simulink model "warning_system"  (R2024b)
settings: Solver=FixedStepAuto  StartTime=0.0  StopTime=inf  FixedStep=TS_MODEL  RelTol=1e-3
InitFcn:
  | %run('config.m');
values from neighbouring files (symbols this model uses):
  ACCEL_RANGE = Simulink.Parameter    [config.m]
  DLPF_SETTING = Simulink.Parameter    [config.m]
  ENABLE_GYRO = Simulink.Parameter    [config.m]
undefined symbols (not defined in the file or in its folder): GYRO_RANGE, THRESHOLD_CAUTION, THRESHOLD_CRASHED, THRESHOLD_LANE_CHANGE, THRESHOLD_REST, TS_CORE, TS_GPS, TS_MPU, TS_PRINT, TS_READER, TS_WRITTER
libraries: arduinolib x5, dspstat3 x3, simulink x3
settings Model: DataDictionary=try.sldd  ExtModeTrigDuration=2  Creator=Nitesh  LastModifiedBy=Nitesh
settings SolverCC: AutoInsertRateTranBlk=on
settings OptimizationCC: EnhancedBackFolding=on  PassReuseOutputArgsAs=Individual arguments  ZeroExternalMemoryAtStartup=off  ZeroInternalMemoryAtStartup=off  MaxStackSize=64  OptimizeBlockOrder=speed  DifferentSizesBufferReuse=on  EfficientTunableParamExpr=on
settings DebuggingCC: ParameterTunabilityLossMsg=error
settings HardwareCC: ProdBitPerPointer=32  ProdBitPerSizeT=32  ProdBitPerPtrDiffT=32  ProdLargestAtomicInteger=Long  ProdLargestAtomicFloat=Double  ProdWordSize=32  ProdHWDeviceType=ARM Compatible->ARM Cortex
settings RTWCC: Description=Embedded Coder  SystemTargetFile=ert.tlc  HardwareBoard=ESP32-WROOM(Arduino Compatible)  TLCOptions="-aInlineSetEventsForThisBaseRateFcn=TLC_FALSE -aSuppressMultiTaskScheduler=TLC_FALSE  -aRateBasedStepFcn=0"  GenCodeOnly=on  PackageGeneratedCodeAndArtifacts=on  TemplateMakefile=ert_default_tmf  Toolchain=ESP32  GenerateCodeMetricsReport=on
settings CodeAppCC: ForceParamTrailComments=on  IgnoreCustomStorageClasses=off  MaxIdLength=51  OperatorAnnotations=on  SimulinkDataObjDesc=on  SFDataObjDesc=on  InsertBlockDesc=on
settings ERTTargetCC: MultiwordLength=2048  DynamicStringBufferSize=2048  InferredTypesCompatibility=on  SupportContinuousTime=on  SupportNonInlinedSFcns=on  SupportVariableSizeSignals=on  ExtModeTransport=3  ExtModeStaticAlloc=on  ExtModeAutomaticAllocSize=off  ExtModeStaticAllocSize=65536  ExtModeMexFile=ext_xcp  ExtModeIntrfLevel=Level2 - Open  InlinedParameterPlacement=Hierarchical

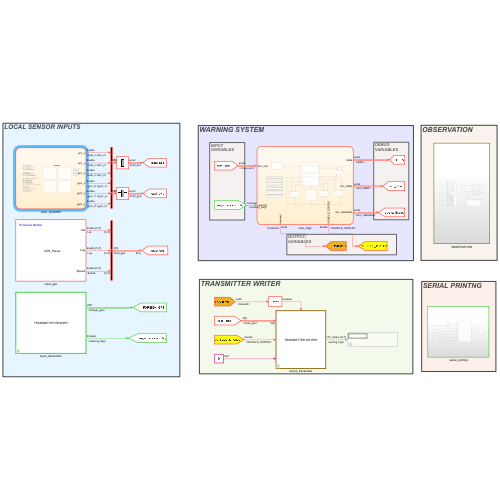
[thumbnail: Simulink's stored preview of the top-level diagram]
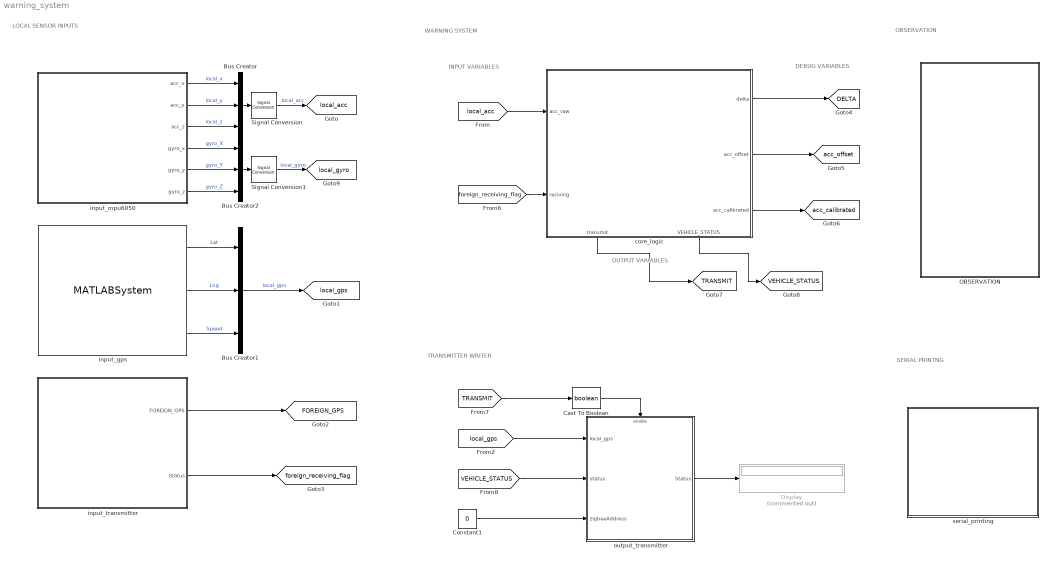
== system warning_system ==
  note: SERIAL PRINTNG
  note: DEBUG
      | VARIABLES
  note: OBSERVATION
  note: TRANSMITTER WRITER
  note: WARNING SYSTEM
  note: LOCAL SENSOR INPUTS
  note: OUTPUT
      | VARIABLES
  note: INPUT
      | VARIABLES
  " serial_printing" : Subsystem
      settings: RTWFileNameOpts=Use subsystem name
  Bus Creator : BusCreator  Inputs=3
  Bus Creator1 : BusCreator  Inputs=3
  Bus Creator2 : BusCreator  Inputs=3
  Cast To Boolean : DataTypeConversion  OutDataTypeStr=boolean  SaturateOnIntegerOverflow=off  RndMeth=Floor
  Constant1 : Constant  Value=0  OutDataTypeStr=half
  Display : Display  Commented=on
  OBSERVATION : Subsystem
  Signal Conversion : SignalConversion  ConversionOutput=Nonvirtual bus  OutDataTypeStr=Bus: accel  OverrideOpt=off
  Signal Conversion1 : SignalConversion  ConversionOutput=Nonvirtual bus  OutDataTypeStr=Bus: accel  OverrideOpt=off
  core_logic : Stateflow chart  TreatAsAtomicUnit=on  SystemSampleTime=TS_CORE
      settings: RTWSystemCode=Reusable function  RTWFileNameOpts=Use subsystem name  PortSchema="{\"entries\":[{\"content\":{\"sides\":[{\"content\":{\"connectorIds\":[\"In2\",\"In1\"]},\"type\":\"ConnectorPlacement.EquallySpacedRectSide\",\"uuid\":\"ee7c9145-97fe-42bf-b38f-25095debb339\"},{\"content\":{\"connectorIds\":[\"Out2\",\"Out3\",\"Out4\"],\"side\":\"RIGHT\"},\"type\":\"ConnectorPlacement.EquallySpacedRectSide\",\"uuid\":\"6ad3cc48-74a8-47e1-8b84-b3331846d199\"},{\"content\":{\"side\":\"TOP\"},\"type\":\"ConnectorPlacement.EquallySpacedRectSide\",\"uuid\":\"0e80e778-40c2-414e-b172-27c343627a22\"},{\"content\":{\"connectorIds\":[\"Out1\",\"Out5\"],\"side\":\"BOTTOM\"},\"type\":\"ConnectorPlacement.EquallySpacedRectSide\",\"uuid\":\"8c076511-fb77-4abd-9a6c-f32e2686fd08\"}]},\"type\":\"ConnectorPlacement.EquallySpacedConnector\",\"uuid\":\"44f6d062-1c8f-4774-b93e-5476bfb914ed\"}],\"packageUris\":[\"http://schema.mathworks.com/mf0/Connector/R2020b\"],\"version\":\"1.0\"}"
  input_gps : MATLABSystem  System=GPS_Parser  SampleTime=TS_GPS
      mask Type: GPS_Parser
      mask Display:
      | color('white');plot([100,100,100,100]*1,[100,100,100,100]*1);plot([100,100,100,100]*0,[100,100,100,100]*0);color('blue');text(38, 92, 'IO Device Builder','horizontalAlignment', 'right');
      | color('black');text(52,50,' GPS_Parser','horizontalAlignment','center');
      | port_label('output',1,'Lat');port_label('output',2,'Lng');port_label('output',3,'Speed');
  input_mpu6050 : Stateflow chart  TreatAsAtomicUnit=on  SystemSampleTime=TS_MPU
      settings: RTWSystemCode=Reusable function  RTWFileNameOpts=Use subsystem name  PortSchema="{\"entries\":[{\"content\":{\"sides\":[{\"content\":{},\"type\":\"ConnectorPlacement.EquallySpacedRectSide\",\"uuid\":\"e0cad0cf-2ed8-4cf7-bff6-6ed2feffa650\"},{\"content\":{\"connectorIds\":[\"Out1\",\"Out3\",\"Out2\",\"Out4\",\"Out5\",\"Out6\"],\"side\":\"RIGHT\"},\"type\":\"ConnectorPlacement.EquallySpacedRectSide\",\"uuid\":\"9c27c799-2435-4d39-8ba1-4c3814f68cde\"},{\"content\":{\"side\":\"TOP\"},\"type\":\"ConnectorPlacement.EquallySpacedRectSide\",\"uuid\":\"52d11aab-2c42-4a19-9ee0-cf61f3e3e234\"}]},\"type\":\"ConnectorPlacement.EquallySpacedConnector\",\"uuid\":\"b37ebc91-bb9d-4b35-9b01-6a26108d89d3\"}],\"packageUris\":[\"http://schema.mathworks.com/mf0/Connector/R2020b\"],\"version\":\"1.0\"}"
  input_transmitter : Subsystem  TreatAsAtomicUnit=on
      settings: RTWFileNameOpts=Use subsystem name
      mask Display: disp('TRANSMITTER READER');
  output_transmitter : Subsystem
      settings: RTWFileNameOpts=Use subsystem name
      mask Display: disp('TRANSMITTER WRITER');
  tag scope: DELTA=global, FOREIGN_GPS=global, TRANSMIT=global, VEHICLE_STATUS=global, acc_calibrated=global, acc_offset=global, foreign_receiving_flag=global, local_acc=global, local_gps=global, local_gyro=global
  wires:
  input_mpu6050/1(acc_x) -> Bus Creator/1  "local_x"
  input_mpu6050/3(acc_y) -> Bus Creator/2  "local_y"
  input_mpu6050/2(acc_z) -> Bus Creator/3  "local_z"
  Bus Creator/1 -> Signal Conversion/1
  [local_acc] -> core_logic/2(acc_raw)
  Bus Creator1/1 -> [local_gps]  "local_gps"
  Constant1/1 -> output_transmitter/3(zigbeeAddress)
  input_transmitter/1(FOREIGN_GPS) -> [FOREIGN_GPS]
  output_transmitter/1(Status) -> Display/1
  input_transmitter/2(Status) -> [foreign_receiving_flag]
  [foreign_receiving_flag] -> core_logic/1(reciving)
  core_logic/2(delta) -> [DELTA]
  core_logic/3(acc_offset) -> [acc_offset]
  core_logic/4(acc_calibrated) -> [acc_calibrated]
  core_logic/5(VEHICLE_STATUS) -> [VEHICLE_STATUS]
  core_logic/1(transmit) -> [TRANSMIT]
  [VEHICLE_STATUS] -> output_transmitter/2(status)
  [TRANSMIT] -> Cast To Boolean/1
  Cast To Boolean/1 -> output_transmitter/Enable
  input_mpu6050/4(gyro_x) -> Bus Creator2/1  "gyro_X"
  input_mpu6050/5(gyro_y) -> Bus Creator2/2  "gyro_Y"
  input_mpu6050/6(gyro_z) -> Bus Creator2/3  "gyro_Z"
  Bus Creator2/1 -> Signal Conversion1/1
  [local_gps] -> output_transmitter/1(local_gps)
  input_gps/1 -> Bus Creator1/1  "Lat"
  input_gps/2 -> Bus Creator1/2  "Lng"
  input_gps/3 -> Bus Creator1/3  "Speed"
  Signal Conversion/1 -> [local_acc]  "local_acc"
  Signal Conversion1/1 -> [local_gyro]  "local_gyro"

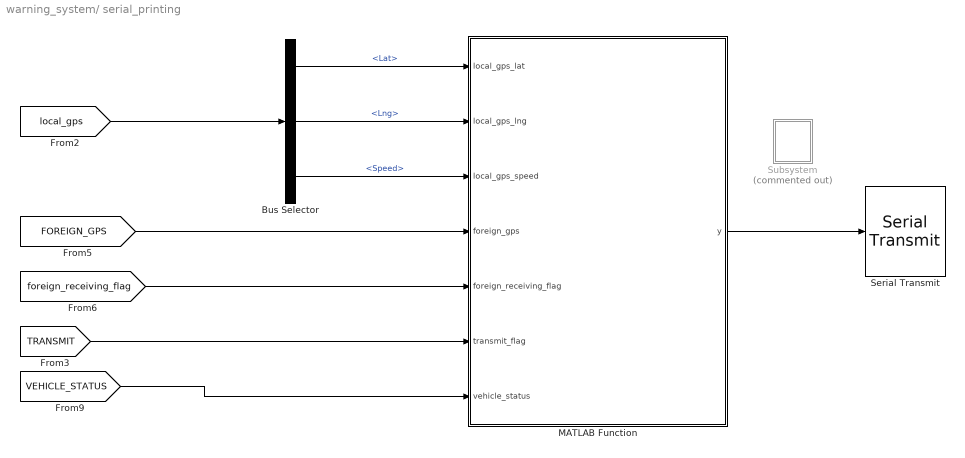
== system warning_system/ serial_printing ==
  Bus Selector : BusSelector  OutputSignals=Lat,Lng,Speed
  MATLAB Function : MATLAB Function  TreatAsAtomicUnit=on  SystemSampleTime=TS_PRINT
  Serial Transmit : arduinolib/Serial Transmit  portNumber=0  sendmode=write  sendformat=Decimal  floatprecision=5  header=[]  terminator=[]  blockPlatform=ARDUINO
      settings: SourceProductName=Common
  Subsystem : Subsystem  Commented=on
  wires:
  MATLAB Function/1(y) -> Serial Transmit/1
  [VEHICLE_STATUS] -> MATLAB Function/7(vehicle_status)
  [TRANSMIT] -> MATLAB Function/6(transmit_flag)
  [FOREIGN_GPS] -> MATLAB Function/4(foreign_gps)
  [local_gps] -> Bus Selector/1
  [foreign_receiving_flag] -> MATLAB Function/5(foreign_receiving_flag)
  Bus Selector/1 -> MATLAB Function/1(local_gps_lat)  "<Lat>"
  Bus Selector/2 -> MATLAB Function/2(local_gps_lng)  "<Lng>"
  Bus Selector/3 -> MATLAB Function/3(local_gps_speed)  "<Speed>"

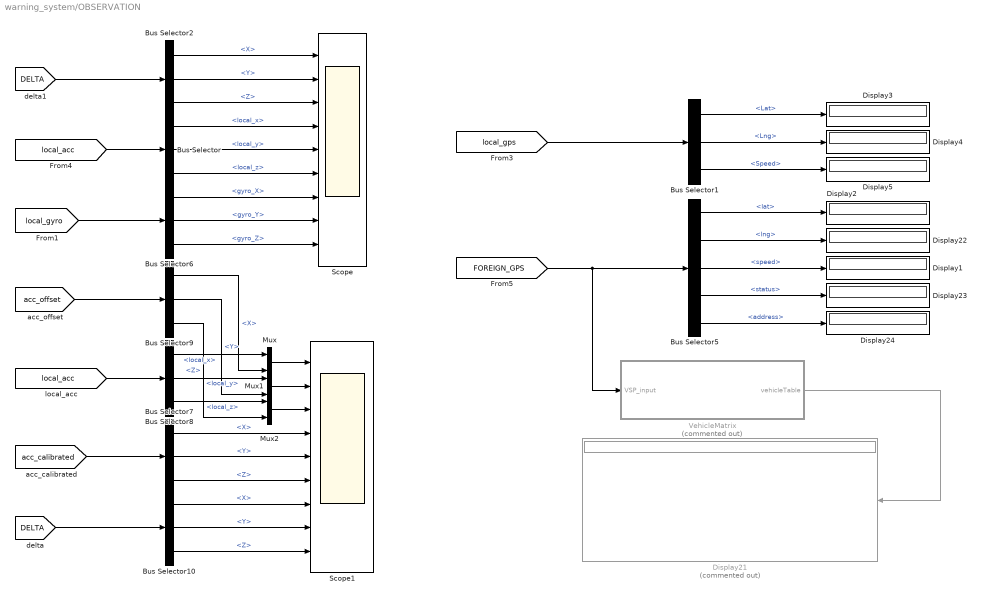
== system warning_system/OBSERVATION ==
  Bus Selector : BusSelector  OutputSignals=local_x,local_y,local_z
  Bus Selector1 : BusSelector  OutputSignals=Lat,Lng,Speed
  Bus Selector{2,7,9..10} (4 alike) : BusSelector  OutputSignals=X,Y,Z
  Bus Selector5 : BusSelector  OutputSignals=lat,lng,speed,status,address
  Bus Selector6 : BusSelector  OutputSignals=gyro_X,gyro_Y,gyro_Z
  Bus Selector8 : BusSelector  OutputSignals=local_x,local_y,local_z
  Display{1..5,22..24} (8 alike) : Display
  Display21 : Display  Commented=on
  Mux : Mux  Inputs=2
  Mux1 : Mux  Inputs=2
  Mux2 : Mux  Inputs=2
  Scope : Scope  NumInputPorts=9
  Scope1 : Scope  NumInputPorts=9
  VehicleMatrix : MATLAB Function  Commented=on  TreatAsAtomicUnit=on
  wires:
  [local_acc] -> Bus Selector/1
  Bus Selector/1 -> Scope/4  "<local_x>"
  Bus Selector/2 -> Scope/5  "<local_y>"
  Bus Selector/3 -> Scope/6  "<local_z>"
  Bus Selector5/1 -> Display2/1  "<lat>"
  Bus Selector5/2 -> Display22/1  "<lng>"
  Bus Selector5/3 -> Display1/1  "<speed>"
  Bus Selector5/4 -> Display23/1  "<status>"
  Bus Selector5/5 -> Display24/1  "<address>"
  VehicleMatrix/1(vehicleTable) -> Display21/1
  [FOREIGN_GPS] -> VehicleMatrix/1(VSP_input), Bus Selector5/1
  Bus Selector6/2 -> Scope/8  "<gyro_Y>"
  Bus Selector6/1 -> Scope/7  "<gyro_X>"
  Bus Selector6/3 -> Scope/9  "<gyro_Z>"
  [local_gyro] -> Bus Selector6/1
  [acc_calibrated] -> Bus Selector7/1
  [local_acc] -> Bus Selector8/1
  [acc_offset] -> Bus Selector9/1
  Mux/1 -> Scope1/1
  Mux2/1 -> Scope1/3
  Bus Selector8/1 -> Mux/1  "<local_x>"
  Bus Selector8/2 -> Mux1/1  "<local_y>"
  Bus Selector8/3 -> Mux2/1  "<local_z>"
  Bus Selector9/1 -> Mux/2  "<X>"
  Bus Selector9/2 -> Mux1/2  "<Y>"
  Bus Selector9/3 -> Mux2/2  "<Z>"
  Mux1/1 -> Scope1/2
  Bus Selector7/1 -> Scope1/4  "<X>"
  Bus Selector7/2 -> Scope1/5  "<Y>"
  Bus Selector7/3 -> Scope1/6  "<Z>"
  [DELTA] -> Bus Selector10/1
  Bus Selector10/1 -> Scope1/7  "<X>"
  Bus Selector10/2 -> Scope1/8  "<Y>"
  Bus Selector10/3 -> Scope1/9  "<Z>"
  [local_gps] -> Bus Selector1/1
  Bus Selector1/3 -> Display5/1  "<Speed>"
  Bus Selector1/1 -> Display3/1  "<Lat>"
  Bus Selector1/2 -> Display4/1  "<Lng>"
  [DELTA] -> Bus Selector2/1
  Bus Selector2/1 -> Scope/1  "<X>"
  Bus Selector2/2 -> Scope/2  "<Y>"
  Bus Selector2/3 -> Scope/3  "<Z>"

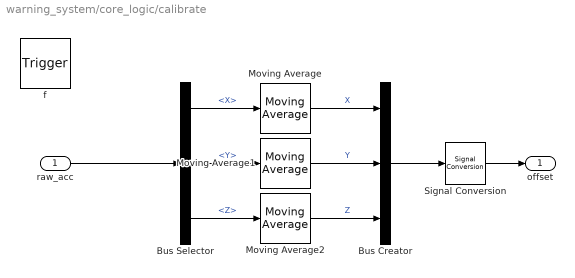
== system warning_system/core_logic/calibrate ==
  raw_acc : Inport  OutDataTypeStr=Bus: accel  PortDimensions=1
  f : TriggerPort  TriggerType=function-call  VariantControl=(inherit)
      settings: CopyFcn=Stateflow.SLINSF.SimulinkMan.removeBlockPreDeleteFcn  PreDeleteFcn=Stateflow.SLINSF.SimulinkMan.unsafePredeleteFcn
  Bus Creator : BusCreator  Inputs=3  OutDataTypeStr=Bus: accel
  Bus Selector : BusSelector  OutputSignals=X,Y,Z
  Moving Average : dspstat3/Moving Average  Method=Sliding window  ForgettingFactorPort=off  SpecifyWindowLength=on  WindowLength=4  OverlapLength=3  AllowArbitraryInputLength=off  ForgettingFactor=0.9  SimulateUsing=Code generation
  Moving Average1 : dspstat3/Moving Average  Method=Sliding window  ForgettingFactorPort=off  SpecifyWindowLength=on  WindowLength=4  OverlapLength=3  AllowArbitraryInputLength=off  ForgettingFactor=0.9  SimulateUsing=Code generation
  Moving Average2 : dspstat3/Moving Average  Method=Sliding window  ForgettingFactorPort=off  SpecifyWindowLength=on  WindowLength=4  OverlapLength=3  AllowArbitraryInputLength=off  ForgettingFactor=0.9  SimulateUsing=Code generation
  Signal Conversion : SignalConversion  ConversionOutput=Nonvirtual bus  OutDataTypeStr=Bus: accel  OverrideOpt=off
  offset : Outport  OutDataTypeStr=Bus: accel
  wires:
  raw_acc/1 -> Bus Selector/1
  Bus Selector/1 -> Moving Average/1  "<X>"
  Bus Selector/2 -> Moving Average1/1  "<Y>"
  Bus Selector/3 -> Moving Average2/1  "<Z>"
  Moving Average/1 -> Bus Creator/1  "X"
  Moving Average1/1 -> Bus Creator/2  "Y"
  Moving Average2/1 -> Bus Creator/3  "Z"
  Bus Creator/1 -> Signal Conversion/1
  Signal Conversion/1 -> offset/1

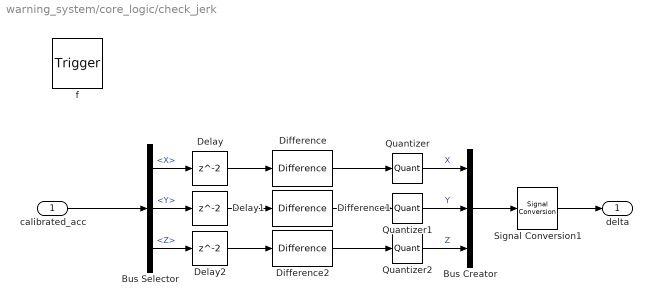
== system warning_system/core_logic/check_jerk ==
  calibrated_acc : Inport  OutDataTypeStr=Bus: accel  PortDimensions=1
  f : TriggerPort  TriggerType=function-call  VariantControl=(inherit)
      settings: CopyFcn=Stateflow.SLINSF.SimulinkMan.removeBlockPreDeleteFcn  PreDeleteFcn=Stateflow.SLINSF.SimulinkMan.unsafePredeleteFcn
  Bus Creator : BusCreator  Inputs=3  OutDataTypeStr=Bus: accel
  Bus Selector : BusSelector  OutputSignals=X,Y,Z
  Delay : Delay
  Delay1 : Delay
  Delay2 : Delay
  Difference : simulink/Discrete/Difference  ICPrevInput=0.0  OutMin=[]  OutMax=[]  OutDataType=fixdt(1, 16)  OutScaling=2^-10  DoSatur=off
  Difference1 : simulink/Discrete/Difference  ICPrevInput=0.0  OutMin=[]  OutMax=[]  OutDataType=fixdt(1, 16)  OutScaling=2^-10  DoSatur=off
  Difference2 : simulink/Discrete/Difference  ICPrevInput=0.0  OutMin=[]  OutMax=[]  OutDataType=fixdt(1, 16)  OutScaling=2^-10  DoSatur=off
  Quantizer : Quantizer  QuantizationInterval=0.1
  Quantizer1 : Quantizer  QuantizationInterval=0.1
  Quantizer2 : Quantizer  QuantizationInterval=0.1
  Signal Conversion1 : SignalConversion  ConversionOutput=Nonvirtual bus  OutDataTypeStr=Bus: accel  OverrideOpt=off
  delta : Outport  OutDataTypeStr=Bus: accel
  wires:
  Delay/1 -> Difference/1
  Difference/1 -> Quantizer/1
  calibrated_acc/1 -> Bus Selector/1
  Bus Selector/1 -> Delay/1  "<X>"
  Quantizer/1 -> Bus Creator/1  "X"
  Quantizer1/1 -> Bus Creator/2  "Y"
  Bus Selector/2 -> Delay1/1  "<Y>"
  Difference1/1 -> Quantizer1/1
  Delay1/1 -> Difference1/1
  Delay2/1 -> Difference2/1
  Difference2/1 -> Quantizer2/1
  Bus Selector/3 -> Delay2/1  "<Z>"
  Quantizer2/1 -> Bus Creator/3  "Z"
  Bus Creator/1 -> Signal Conversion1/1
  Signal Conversion1/1 -> delta/1

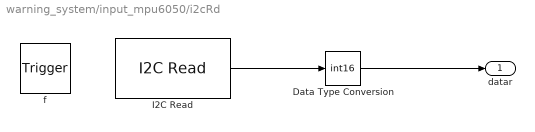
== system warning_system/input_mpu6050/i2cRd ==
  f : TriggerPort  TriggerType=function-call  VariantControl=Variant  SampleTime=inf
      settings: CopyFcn=Stateflow.SLINSF.SimulinkMan.removeBlockPreDeleteFcn  PreDeleteFcn=Stateflow.SLINSF.SimulinkMan.unsafePredeleteFcn
  Data Type Conversion : DataTypeConversion  OutDataTypeStr=int16  SaturateOnIntegerOverflow=off  RndMeth=Floor
  I2C Read : arduinolib/I2C Read  I2CModule=0  Mode=Master  SlaveAddress=hex2dec( '68' )  SlaveByteOrder=BigEndian  Direction=Receiver  RegisterAddressMode=on  RegisterAddress=hex2dec( '3b' )  SlaveDataType=uint16  DataLength=7  NoAck=off  RepeatedStart=off  OutputStatus=off  blockPlatform=arduino  SampleTime=-1
      settings: SourceProductName=Common
  datar : Outport  Unit=1  VectorParamsAs1DForOutWhenUnconnected=off
  wires:
  I2C Read/1 -> Data Type Conversion/1
  Data Type Conversion/1 -> datar/1

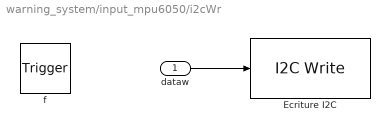
== system warning_system/input_mpu6050/i2cWr ==
  dataw : Inport  OutDataTypeStr=uint16  Unit=1  PortDimensions=1
  f : TriggerPort  TriggerType=function-call  VariantControl=Variant  SampleTime=-1
      settings: CopyFcn=Stateflow.SLINSF.SimulinkMan.removeBlockPreDeleteFcn  PreDeleteFcn=Stateflow.SLINSF.SimulinkMan.unsafePredeleteFcn
  Ecriture I2C : arduinolib/I2C Write  Priority=1  I2CModule=0  Mode=Master  SlaveAddress=hex2dec( '68' )  SlaveByteOrder=BigEndian  Direction=Transmitter  RegisterAddressMode=off  RegisterAddress=hex2dec( '6B' )  SlaveDataType=uint16  DataLength=1  NoAck=off  RepeatedStart=off  OutputStatus=off  blockPlatform=arduino
      settings: SourceProductName=Common
  wires:
  dataw/1 -> Ecriture I2C/1

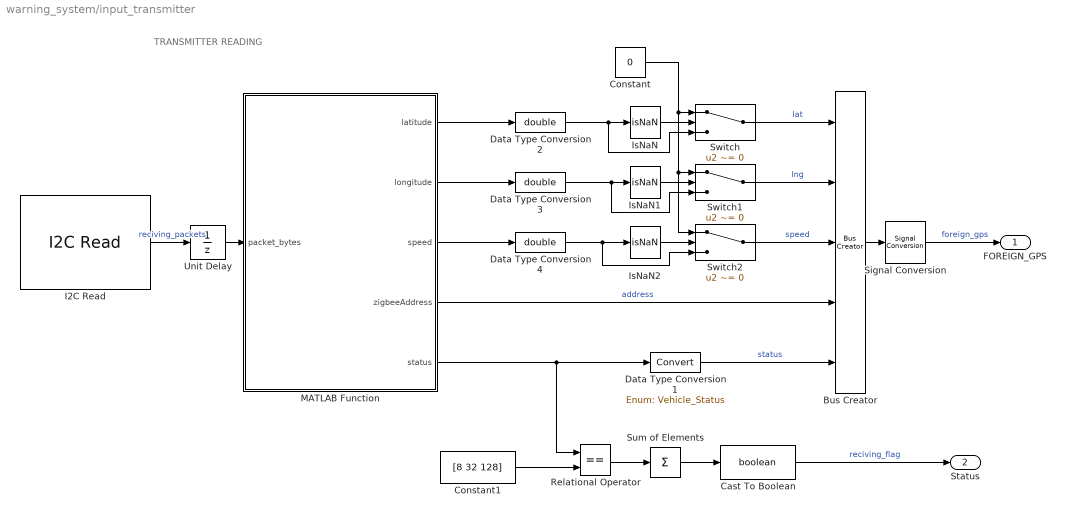
== system warning_system/input_transmitter ==
  note: TRANSMITTER READING
  Bus Creator : BusCreator  Inputs=5  OutDataTypeStr=Bus: VSP
  Cast To Boolean : DataTypeConversion  OutDataTypeStr=boolean  SaturateOnIntegerOverflow=off  RndMeth=Floor
  Constant : Constant  Value=0  OutDataTypeStr=double
  Constant1 : Constant  Value=[8 32 128]
  Data Type Conversion1 : DataTypeConversion  OutDataTypeStr=Enum: Vehicle_Status  SaturateOnIntegerOverflow=off  RndMeth=Floor
  Data Type Conversion2 : DataTypeConversion  OutDataTypeStr=double  SaturateOnIntegerOverflow=off  RndMeth=Floor
  Data Type Conversion3 : DataTypeConversion  OutDataTypeStr=double  SaturateOnIntegerOverflow=off  RndMeth=Floor
  Data Type Conversion4 : DataTypeConversion  OutDataTypeStr=double  SaturateOnIntegerOverflow=off  RndMeth=Floor
  I2C Read : arduinolib/I2C Read  I2CModule=0  Mode=Master  SlaveAddress=hex2dec('3C')  SlaveByteOrder=BigEndian  Direction=Receiver  RegisterAddressMode=off  RegisterAddress=0  SlaveDataType=uint8  DataLength=15  NoAck=off  RepeatedStart=off  OutputStatus=off  blockPlatform=ARDUINO  SampleTime=TS_READER
      settings: SourceProductName=Common
  IsNaN : RelationalOperator  Operator=isNaN  OutDataTypeStr=boolean  RndMeth=Simplest  InputSameDT=off
  IsNaN1 : RelationalOperator  Operator=isNaN  OutDataTypeStr=boolean  RndMeth=Simplest  InputSameDT=off
  IsNaN2 : RelationalOperator  Operator=isNaN  OutDataTypeStr=boolean  RndMeth=Simplest  InputSameDT=off
  MATLAB Function : MATLAB Function  TreatAsAtomicUnit=on
  Relational Operator : RelationalOperator  Operator===  OutDataTypeStr=boolean  RndMeth=Simplest  InputSameDT=off
  Signal Conversion : SignalConversion  ConversionOutput=Nonvirtual bus  OutDataTypeStr=Bus: VSP  OverrideOpt=off
  Sum of Elements : Sum  Inputs=+
  Switch : Switch  Criteria=u2 ~= 0  SaturateOnIntegerOverflow=off  InputSameDT=off
  Switch1 : Switch  Criteria=u2 ~= 0  SaturateOnIntegerOverflow=off  InputSameDT=off
  Switch2 : Switch  Criteria=u2 ~= 0  SaturateOnIntegerOverflow=off  InputSameDT=off
  Unit Delay : UnitDelay  SampleTime=-1  HasFrameUpgradeWarning=on
  FOREIGN_GPS : Outport  OutDataTypeStr=Bus: VSP
  Status : Outport  Port=2  OutDataTypeStr=boolean
  wires:
  I2C Read/1 -> Unit Delay/1  "reciving_packets"
  MATLAB Function/1(latitude) -> Data Type Conversion2/1
  MATLAB Function/2(longitude) -> Data Type Conversion3/1
  MATLAB Function/3(speed) -> Data Type Conversion4/1
  MATLAB Function/5(status) -> Data Type Conversion1/1, Relational Operator/1
  MATLAB Function/4(zigbeeAddress) -> Bus Creator/4  "address"
  Bus Creator/1 -> Signal Conversion/1
  Unit Delay/1 -> MATLAB Function/1(packet_bytes)
  Data Type Conversion1/1 -> Bus Creator/5  "status"
  Signal Conversion/1 -> FOREIGN_GPS/1  "foreign_gps"
  Relational Operator/1 -> Sum of Elements/1
  Constant1/1 -> Relational Operator/2
  Sum of Elements/1 -> Cast To Boolean/1
  Cast To Boolean/1 -> Status/1  "reciving_flag"
  Switch/1 -> Bus Creator/1  "lat"
  Switch1/1 -> Bus Creator/2  "lng"
  Switch2/1 -> Bus Creator/3  "speed"
  IsNaN/1 -> Switch/2
  Data Type Conversion2/1 -> Switch/3, IsNaN/1
  Data Type Conversion3/1 -> Switch1/3, IsNaN1/1
  Data Type Conversion4/1 -> Switch2/3, IsNaN2/1
  IsNaN1/1 -> Switch1/2
  IsNaN2/1 -> Switch2/2
  Constant/1 -> Switch2/1, Switch1/1, Switch/1

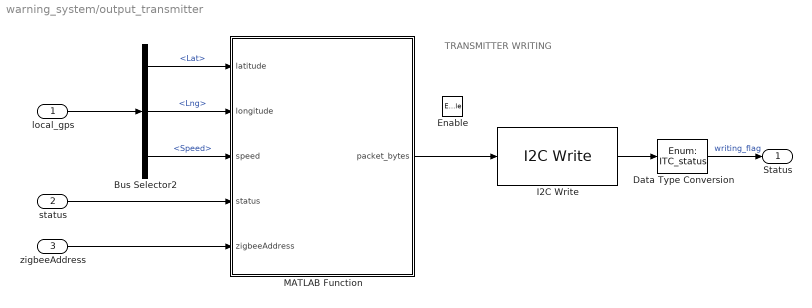
== system warning_system/output_transmitter ==
  note: TRANSMITTER WRITING
  local_gps : Inport
  status : Inport  Port=2
  zigbeeAddress : Inport  Port=3
  Enable : EnablePort
  Bus Selector2 : BusSelector  OutputSignals=Lat,Lng,Speed
  Data Type Conversion : DataTypeConversion  OutDataTypeStr=Enum: ITC_status  SaturateOnIntegerOverflow=off  RndMeth=Floor
  I2C Write : arduinolib/I2C Write  I2CModule=0  Mode=Master  SlaveAddress=hex2dec('3C')  SlaveByteOrder=BigEndian  Direction=Transmitter  RegisterAddressMode=off  RegisterAddress=0  SlaveDataType=uint8  DataLength=1  NoAck=off  RepeatedStart=off  OutputStatus=on  blockPlatform=ARDUINO
      settings: SourceProductName=Common
  MATLAB Function : MATLAB Function  TreatAsAtomicUnit=on  SystemSampleTime=TS_WRITTER
  Status : Outport
  wires:
  MATLAB Function/1(packet_bytes) -> I2C Write/1
  I2C Write/1 -> Data Type Conversion/1
  zigbeeAddress/1 -> MATLAB Function/5(zigbeeAddress)
  local_gps/1 -> Bus Selector2/1
  status/1 -> MATLAB Function/4(status)
  Data Type Conversion/1 -> Status/1  "writing_flag"
  Bus Selector2/1 -> MATLAB Function/1(latitude)  "<Lat>"
  Bus Selector2/2 -> MATLAB Function/2(longitude)  "<Lng>"
  Bus Selector2/3 -> MATLAB Function/3(speed)  "<Speed>"

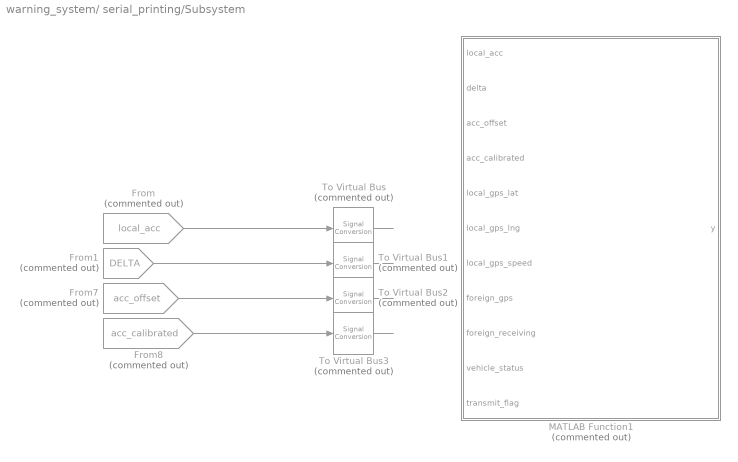
== system warning_system/ serial_printing/Subsystem ==
  From : From  Commented=on  GotoTag=local_acc  TagVisibility=global
  From1 : From  Commented=on  GotoTag=DELTA  TagVisibility=global
  From7 : From  Commented=on  GotoTag=acc_offset  TagVisibility=global
  From8 : From  Commented=on  GotoTag=acc_calibrated  TagVisibility=global
  MATLAB Function1 : MATLAB Function  Commented=on  TreatAsAtomicUnit=on  SystemSampleTime=TS_PRINT
  To Virtual Bus{,1..3} (4 alike) : SignalConversion  Commented=on  ConversionOutput=Nonvirtual bus  OutDataTypeStr=Bus: accel  OverrideOpt=off
  wires:
  To Virtual Bus3/1 -> ?
  From/1 -> To Virtual Bus/1
  From8/1 -> To Virtual Bus3/1
  To Virtual Bus2/1 -> ?
  From1/1 -> To Virtual Bus1/1
  From7/1 -> To Virtual Bus2/1
  To Virtual Bus1/1 -> ?
  To Virtual Bus/1 -> ?

== stateflow chart warning_system/input_mpu6050 ==
  note: MPU6050
  note: Accelerometer Configuration
      | Register: 0x1C (ACCEL_CONFIG)
      | 0x00 → ±2g (highest sensitivity, lowest range)
      | 0x08 → ±4g (moderate sensitivity)
      | 0x10 → ±8g (lower sensitivity, higher range)
      | 0x18 → ±16g (lowest sensitivity, highest range)
      | Gyroscope Configuration
      | Register: 0x1B (GYRO_CONFIG)
      | 0x00 → ±250°/s (highest sensitivity, lowest range)
      | 0x08 → ±500°/s (moderate sensitivity)
      | 0x10 → ±1000°/s (lower sensitivity, higher range)
      | 0x18 → ±2000°/s (lowest sensitivity, highest range)
      | Digital Low-Pass Filter (DLPF) and Update Rate
      | Register: 0x1A (CONFIG)
      | 0x00 → 260Hz bandwidth, 0ms delay
      | 0x01 → 184Hz bandwidth, 2.0ms delay
      | 0x02 → 94Hz bandwidth, 3.0ms delay
      | 0x03 → 44Hz bandwidth, 4.9ms delay
      | 0x04 → 21Hz bandwidth, 8.5ms delay
      | 0x05 → 10Hz bandwidth, 13.8ms delay
      | 0x06 → 5Hz bandwidth, 19.0ms delay (lowest noise, highest filtering)
      | Power Management
      | Register: 0x6B (PWR_MGMT_1)
      | 0x00 → Wake up device, use internal 8MHz oscillator
      | Register: 0x6C (PWR_MGMT_2)
      | 0x07 → Disable all gyroscope axes (X, Y, Z)
      | 0x00 → Enable all gyroscope axes
  state Initialisation
    en:
    % -------------- Power Management --------------
    i2cWr(uint16(hex2dec('6B00'))); % Power on
    % Check if Gyroscope should be disabled
    if ~ENABLE_GYRO
    i2cWr(uint16(hex2dec('6C07'))); % Disable Gyroscope
    else
    i2cWr(uint16(hex2dec('6C00'))); % Enable Gyroscope
    end
    % -------------- Digital Low-Pass Filter --------------
    if DLPF_SETTING >= 0 && DLPF_SETTING <= 6
    i2cWr(uint16(0x1A00) + uint16(DLPF_SETTING));
    else
    error('Invalid DLPF setting');
    end
    disp('MPU6050 Initialization Completed.');
  state MPU_Running
    during:
    % Read raw data from MPU6050
    val = i2cRd;
    % Extract acceleration values (X, Y, Z)
    raw_acc_x=val(1);
    raw_acc_y=val(2);
    raw_acc_z=val(3);
    temp = (double(val(4))/340.0) +36.53;
    raw_gryo_x = val(5);
    raw_gryo_y = val(6);
    raw_gryo_z = val(7);
    %
    acc_x = double(raw_acc_x) / double(acc_scale_factor);
    acc_y = double(raw_acc_y) / double(acc_scale_factor);
    acc_z = double(raw_acc_z) / double(acc_scale_factor);
    %
    gyro_x = double(raw_gryo_x) / double(gyro_scale_factor);
    gyro_y = double(raw_gryo_y) / double(gyro_scale_factor);
    gyro_z = double(raw_gryo_z) / double(gyro_scale_factor);
  state datar = i2cRd [function]
  state i2cWr(dataw) [function]
  state Accelerometer_Configuration
    en:
    switch ACCEL_RANGE
    case uint8(2)
    i2cWr(uint16(0x1C00));
    acc_scale_factor = 16384;  % ±2g
    case uint8(4)
    i2cWr(uint16(0x1C08));
    acc_scale_factor = 8192;   % ±4g
    case uint8(8)
    i2cWr(uint16(0x1C10));
    acc_scale_factor = 4096;   % ±8g
    case uint8(16)
    i2cWr(uint16(0x1C18));
    acc_scale_factor = 2048;   % ±16g
    otherwise
    error('Invalid Accelerometer Range');
    end
  state Gyro_Configuration
    en:
    switch GYRO_RANGE
    case 250
    i2cWr(uint16(0x1B00));
    gyro_scale_factor = 131;  % ± 250 °/s
    case 500
    i2cWr(uint16(0x1B08));
    gyro_scale_factor = 65.5;   % ± 500 °/s
    case 1000
    i2cWr(uint16(0x1B10));
    gyro_scale_factor = 32.2;   % ± 1000 °/s
    case 2000
    i2cWr(uint16(0x1B18));
    gyro_scale_factor = 16.4;   % ± 2000 °/s
    otherwise
    error('Invalid Gyro Range');
    end
  (default) -> Initialisation
  Initialisation -> Accelerometer_Configuration
  Gyro_Configuration -> MPU_Running
  Accelerometer_Configuration -> Gyro_Configuration
  data: datar function_output; dataw function_input uint16 size=1; val local int16 size=7; acc_x output double; acc_z output double; acc_y output double; raw_acc_x local int16; raw_acc_y local int16; raw_acc_z local int16; ENABLE_GYRO parameter double; ACCEL_RANGE parameter uint8; DLPF_SETTING parameter double; GYRO_RANGE parameter; raw_gryo_x local; raw_gryo_y local; raw_gryo_z local; gyro_scale_factor local double; acc_scale_factor local; temp local; gyro_x output; gyro_y output; gyro_z output

== matlab function warning_system/output_transmitter/MATLAB Function ==
  data: latitude input; packet_bytes output; longitude input; speed input; status input; zigbeeAddress input
function packet_bytes = create_i2c_packet(latitude, longitude, speed, status, zigbeeAddress)
    %#codegen

    % Define fixed-size output (1x15 uint8 array)
    packet_bytes = zeros(1, 15, 'uint8'); 

    % single --> float32
    % double --> float64

    % Convert to byte representation
    lat_bytes = typecast(single(latitude), 'uint8'); % 4 byte
    lon_bytes = typecast(single(longitude), 'uint8'); % 4 byte
    speed_bytes = typecast(single(speed), 'uint8'); % 4 byte
    status_byte = uint8(status); % 1 byte
    zigbee_bytes = typecast(uint16(zigbeeAddress), 'uint8'); % 2 bytes 

    % Store in the output array
    packet_bytes(1:4)   = lat_bytes;
    packet_bytes(5:8)   = lon_bytes;
    packet_bytes(9:12)  = speed_bytes;
    packet_bytes(13:14) = zigbee_bytes;
    packet_bytes(15)    = status_byte; % Adjusted for uint32
end

== matlab function warning_system/ serial_printing/Subsystem/MATLAB Function1 ==
  data: y output uint8 size=[1 600]; local_acc input; delta input; acc_offset input; acc_calibrated input; local_gps_lat input; local_gps_lng input; local_gps_speed input; foreign_gps input; foreign_receiving input; vehicle_status input; transmit_flag input
function y = formatVehicleData( ...
    local_acc, delta, acc_offset, acc_calibrated, ...
    local_gps_lat, local_gps_lng, local_gps_speed, ...
    foreign_gps, ...
    foreign_receiving, vehicle_status, ...
    transmit_flag)
%#codegen

    % Pre-allocate fixed-size output (600 bytes)
    y = zeros(1, 600, 'uint8');  % fixed 600-byte output
    str = blanks(600);           % pre-fill with 600 spaces (char array)

    % Force logicals to int
    txFlag = int32(transmit_flag);
    % rxFlag = int32(receiving_flag);
    foreign_receiving = int32(foreign_receiving);
    vehicle_status = int32(vehicle_status);

    switch vehicle_status
        case 0
            statusStr = 'INVALID';
        case 4
            statusStr = 'NORMAL';
        case 8
            statusStr = 'LANE_CHANGE_RIGHT';
        case 16
            statusStr = 'LANE_CHANGE_LEFT';
        case 32
            statusStr = 'NEARBY_CRASH';
        case 128
            statusStr = 'CRASH';
        otherwise
            statusStr = 'UNKNOWN';
    end

    % Format the message string
    formatted = sprintf([ ...
        '----------------\n', ...
        'INFORMATION\n', ...
        '----------------\n', ...
        'Local Acc:         (%.6f, %.6f, %.6f)\n', ...
        'Delta:             (%.2f, %.2f, %.2f)\n', ...
        'Offset:            (%.3f, %.3f, %.3f)\n', ...
        'Calibrated Acc:    (%.6f, %.6f, %.6f)\n', ...
        'Local GPS:         (%.7f, %.7f) , Speed=%.2f\n', ...
        'Foreign GPS:       (%.7f, %.7f) , Speed=%.2f\n', ...
        'Foreign RECEIVING:  %d\n', ...
        'Vehicle Status:     %d (%s)\n', ...
        'TRANSMITTING Flag:  %d\n', ...
        '\n'], ...
        local_acc.X, local_acc.Y, local_acc.Z, ...
        delta.X, delta.Y, delta.Z, ...
        acc_offset.X, acc_offset.Y, acc_offset.Z, ...
        acc_calibrated.X, acc_calibrated.Y, acc_calibrated.Z, ...
        local_gps_lat, local_gps_lng, local_gps_speed, ...
        foreign_gps.lat, foreign_gps.lng, foreign_gps.speed, ...
        foreign_receiving, ...
        vehicle_status, statusStr,...
        txFlag);

    % Copy characters into the fixed-length string
    len = min(length(formatted), 600);
    str(1:len) = formatted(1:len);

    % Convert to uint8 for output
    y = uint8(str);
end

== matlab function warning_system/input_transmitter/MATLAB Function ==
  data: packet_bytes input; latitude output; longitude output; speed output; zigbeeAddress output; status output
function [latitude, longitude, speed, zigbeeAddress, status] = read_i2c_packet(packet_bytes)
    %#codegen

    % Define output sizes and types
    latitude = single(0);
    longitude = single(0);
    speed = single(0);
    status = uint8(0);
    zigbeeAddress = uint16(0);

    % Validate packet size
    if length(packet_bytes) ~= 15
        return; % Return default values if packet size is incorrect
    end

    % Extract byte segments and convert back to original data types
    latitude = typecast(uint8(packet_bytes(1:4)), 'single');
    longitude = typecast(uint8(packet_bytes(5:8)), 'single');
    speed = typecast(uint8(packet_bytes(9:12)), 'single');
    zigbeeAddress = typecast(uint8(packet_bytes(13:14)), 'uint16'); % Reconstruct as uint16
    status = uint8(packet_bytes(15)); % Already uint8, no need for typecast
end

== matlab function warning_system/ serial_printing/MATLAB Function ==
  data: y output uint8 size=[1 130]; local_gps_lat input; local_gps_lng input; local_gps_speed input; foreign_gps input; foreign_receiving_flag input; transmit_flag input; vehicle_status input
function y = formatVehicleData( ...
    local_gps_lat, local_gps_lng, local_gps_speed, foreign_gps, ...
    foreign_receiving_flag, transmit_flag, ...
    vehicle_status)
    %#codegen

    % Pre-allocate fixed-size output (600 bytes)
    y = zeros(1, 130, 'uint8');  % fixed 600-byte output
    str = blanks(130);           % pre-fill with 600 spaces (char array)

    % Force logicals to int
    transmit_flag = int32(transmit_flag);
    foreign_receiving_flag = int32(foreign_receiving_flag);
    vehicle_status = int32(vehicle_status);

    switch vehicle_status
        case 0
            statusStr = 'INVALID';
        case 4
            statusStr = 'NORMAL';
        case 8
            statusStr = 'LANE_CHANGE_RIGHT';
        case 16
            statusStr = 'LANE_CHANGE_LEFT';
        case 32
            statusStr = 'NEARBY_CRASH';
        case 128
            statusStr = 'CRASH';
        case 100
            statusStr = 'CAUTION';
        otherwise
            statusStr = 'UNKNOWN';
    end

    % Format the message string
    formatted = sprintf([ '\n<%17s (%3d) || TRANSMIT: %2d || (%.7f, %.7f, %.3f) || RECEIVING: %d || (%.7f, %.7f, %.3f)>'], ...
    statusStr, vehicle_status, ...
    transmit_flag, local_gps_lat, local_gps_lng, local_gps_speed, ...
    foreign_receiving_flag , foreign_gps.lat, foreign_gps.lng, foreign_gps.speed ...
    );
    % Copy characters into the fixed-length string
    len = min(length(formatted), 130);
    str(1:len) = formatted(1:len);

    % Convert to uint8 for output
    y = uint8(str);
end

== stateflow chart warning_system/core_logic ==
  state Init
    en:
    COUNT_CALIBRATION = 10;
    VEHICLE_STATUS=8;
    COUNT_CRASHED=0;
    COUNT_NEARBY_CRASHED=0;
    COUNT_CAUTION=0;
    transmit = 0;
  state mpu_running
    state extracting_acc
      during:
      acc_calibrated.X =  acc_raw.X - acc_offset.X;
      acc_calibrated.Y =  acc_raw.Y - acc_offset.Y;
      acc_calibrated.Z =  acc_raw.Z - acc_offset.Z;
    state delta_computation
      en:
      delta = check_jerk(acc_calibrated);
    (default) -> extracting_acc
    extracting_acc -> delta_computation [order 3] : [temporalCount(tick)>1]
  state caliberation
    en:
    acc_offset =   calibrate(acc_raw);
  state NORMAL
    entry:
    VEHICLE_STATUS=4;
    if (transmit>0)
    transmit = transmit-1;
    end
    if (lane_changed==1)
    %RIGHT
    VEHICLE_STATUS =8;
    transmit = 8;
    elseif (lane_changed==-1)
    %LEFT
    VEHICLE_STATUS =16;
    transmit = 8;
    end
  state delta = check_jerk(calibrated_acc) [function]
  state CAUTION
    en:
    VEHICLE_STATUS=100;
  state CRASHED
    entry:
    VEHICLE_STATUS=128;
  state NEARBY_CRASH
    entry:
    VEHICLE_STATUS=32;
  state offset = calibrate(raw_acc) [function]
  (default) -> Init
  Init -> mpu_running
  extracting_acc -> (junction 43) [order 1] : [is_rest && offset_mismatch(COUNT_CALIBRATION)]
  (junction 43) -> caliberation
  extracting_acc -> (junction 40) [order 2] : [COUNT_CALIBRATION>0]
      | {COUNT_CALIBRATION = COUNT_CALIBRATION - 1}
  (junction 40) -> caliberation
  caliberation -> (junction 35)
  (junction 35) -> mpu_running
  (junction 103) -> mpu_running
  (junction 102) -> (junction 103)
  delta_computation -> (junction 142) [order 3] : [COUNT_CRASHED>4]
  (junction 142) -> CRASHED
  delta_computation -> (junction 145) [order 2] : [is_crashed]
  (junction 145) -> CRASHED : {COUNT_CRASHED = 15;}
  delta_computation -> (junction 154) [order 4] : [COUNT_NEARBY_CRASHED>10]
  (junction 154) -> NEARBY_CRASH
  delta_computation -> (junction 167) [order 6] : [COUNT_CAUTION>5]
  delta_computation -> (junction 148) [order 1] : [reciving==true]
  (junction 167) -> CAUTION
  delta_computation -> (junction 181) [order 5]
  (junction 148) -> NEARBY_CRASH : {COUNT_NEARBY_CRASHED = 8}
  (junction 181) -> CAUTION : [is_caution]
      | {COUNT_CRASHED=7}
  delta_computation -> NORMAL [order 7]
  CAUTION -> (junction 161) : {
      | COUNT_CAUTION = COUNT_CAUTION-1;
      | transmit=COUNT_CAUTION;
      | }
  CRASHED -> (junction 97) : {
      | COUNT_CRASHED = COUNT_CRASHED-1;
      | transmit=COUNT_CRASHED;
      | }
  NEARBY_CRASH -> (junction 93) : {
      | COUNT_NEARBY_CRASHED = COUNT_NEARBY_CRASHED-1
      | transmit = COUNT_NEARBY_CRASHED
      | }
  NORMAL -> (junction 96)
  (junction 93) -> (junction 102)
  (junction 96) -> (junction 93)
  (junction 161) -> (junction 96)
  (junction 97) -> (junction 161)
  data: COUNT_CALIBRATION function_input; count function_output; y function_output; y function_output; y function_output; y function_output; calibrated_acc function_input Bus: accel size=1; delta function_output Bus: accel; raw_acc function_input Bus: accel size=1; offset function_output Bus: accel; transmit output uint8; reciving input boolean; COUNT_CALIBRATION local uint8; THRESHOLD_REST parameter; THRESHOLD_CRASHED parameter; delta output Bus: accel size=1 =struct('X', 0, 'Y', 0, 'Z', 0); acc_offset output Bus: accel size=1 =struct('X', 0, 'Y', 0, 'Z', 0); acc_calibrated output Bus: accel size=1 =struct('X', 0, 'Y', 0, 'Z', 0); acc_raw input Bus: accel; VEHICLE_STATUS output; COUNT_CRASHED local uint8; COUNT_NEARBY_CRASHED local uint8; THRESHOLD_CAUTION parameter; THRESHOLD_LANE_CHANGE parameter; COUNT_CAUTION local uint8
  function count = offset_mismatch(COUNT_CALIBRATION):
    | function count = offset_mismatch(COUNT_CALIBRATION)
    | 
    | count = COUNT_CALIBRATION;
    | if(abs(acc_raw.X - acc_offset.X) > 0.01 && ...
    |    abs(acc_raw.Y - acc_offset.Y) > 0.01 && ...
    |    abs(acc_raw.Z - acc_offset.Z) > 0.01)
    | 
    |     count = COUNT_CALIBRATION +1;
    | end
  function y = lane_changed:
    | function y = lane_changed
    | 
    | y = 0;
    | 
    | if (acc_calibrated.X > THRESHOLD_LANE_CHANGE)
    |     % LEFT
    |     y = 1; 
    | elseif (acc_calibrated.X < -THRESHOLD_LANE_CHANGE)
    |     % RIGHT
    |     y = -1;
    | end
  function y = is_caution:
    | function y = is_caution
    |  
    | 
    | if (abs(delta.Y) >= THRESHOLD_CAUTION)
    |    
    |     y = true; 
    | else 
    |     y = false;
    | end
  function y = is_rest:
    | function y = is_rest
    | 
    | if (abs(delta.X) >= THRESHOLD_REST &&...
    |     abs(delta.Y) >= THRESHOLD_REST &&...
    |     abs(delta.Z) >= THRESHOLD_REST )
    |     y = true; 
    | else 
    |     y = false;
    | end
  function y = is_crashed:
    | function y = is_crashed
    | 
    | if (abs(delta.Y) >= THRESHOLD_CRASHED)
    |     y = true; 
    | else 
    |     y = false;
    | end

== matlab function warning_system/OBSERVATION/VehicleMatrix ==
  data: VSP_input input; vehicleTable output size=[10, 5]
function vehicleTable = updateVehicleMatrix(VSP_input)
    %#codegen
    persistent table
    maxRows = 10;
    numCols = 5;

    if isempty(table)
        table = zeros(maxRows, numCols);  % Fixed size [10x5]
    end

    % Predeclare output for fixed-size requirement
    vehicleTable = zeros(maxRows, numCols);

    % Check if vehicle already exists — update if found
    for i = 1:maxRows
        if table(i, 1) == double(VSP_input.address)
            table(i, :) = [ ...
                double(VSP_input.address), ...
                double(VSP_input.status), ...
                VSP_input.lat, ...
                VSP_input.lng, ...
                VSP_input.speed];
            vehicleTable = table;
            return;
        end
    end

    % Try to insert into first empty row
    for i = 1:maxRows
        if table(i, 1) == 0
            table(i, :) = [ ...
                double(VSP_input.address), ...
                double(VSP_input.status), ...
                VSP_input.lat, ...
                VSP_input.lng, ...
                VSP_input.speed];
            vehicleTable = table;
            return;
        end
    end

    % If full, replace first row
    table(1, :) = [ ...
        double(VSP_input.address), ...
        double(VSP_input.status), ...
        VSP_input.lat, ...
        VSP_input.lng, ...
        VSP_input.speed];

    vehicleTable = table;
end
